simulink model "Mass_Spring_Damper"  (R2022b)
settings: Solver=VariableStepAuto  StartTime=0.0  StopTime=10.0  MaxStep=1e-3  RelTol=1e-3
values from neighbouring files (symbols this model uses):
  b = 10    [MassSpringDamper.m]
  k = 400    [MassSpringDamper.m]
  m = massValue(i)    [MassSpringDamper.m]
  x0 = 1    [MassSpringDamper.m]
settings Model: Creator=NourAldin  LastModifiedBy=NourAldin

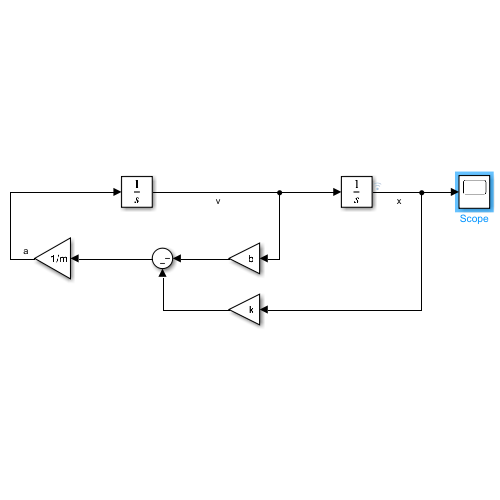
[thumbnail: Simulink's stored preview of the top-level diagram]
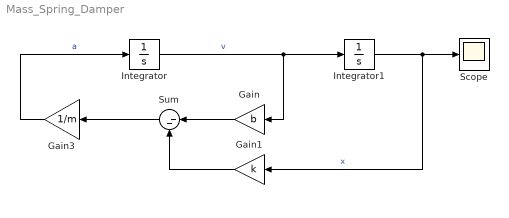
== system Mass_Spring_Damper ==
  Gain : Gain  Gain=b
  Gain1 : Gain  Gain=k
  Gain3 : Gain  Gain=1/m
  Integrator : Integrator
  Integrator1 : Integrator  InitialCondition=x0
  Scope : Scope
  Sum : Sum  Inputs=|--
  wires:
  Integrator/1 -> Integrator1/1, Gain/1  "v"
  Integrator1/1 -> Scope/1, Gain1/1  "x"
  Gain/1 -> Sum/1
  Gain1/1 -> Sum/2
  Sum/1 -> Gain3/1
  Gain3/1 -> Integrator/1  "a"
